simulink library "imu_block"  (R2025b)
settings: Solver=VariableStepAuto  StartTime=0.0  StopTime=10.0  RelTol=1e-3
values from neighbouring files (symbols this model uses):
  IMU_T03 = casper_imu_local_params()    [test_imu_model.m]
undefined symbols (not defined in the file or in its folder): ADXL, Attitude, Estimator, IMU, Sim
settings Model: Creator=Ashwin  LastModifiedBy=Ashwin

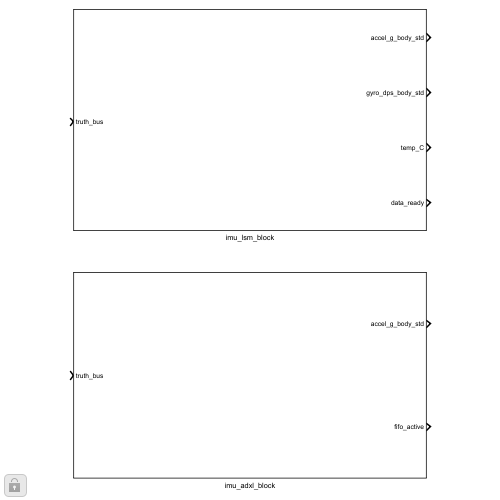
[thumbnail: Simulink's stored preview of the top-level diagram]
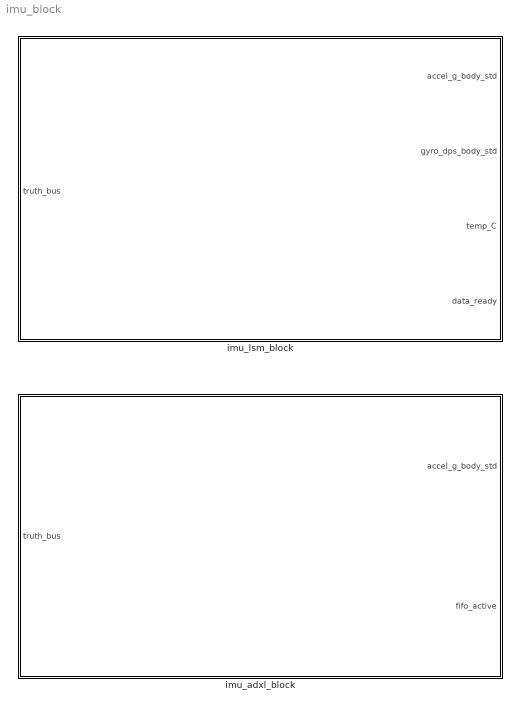
== system imu_block ==
  imu_adxl_block : Subsystem
  imu_lsm_block : Subsystem

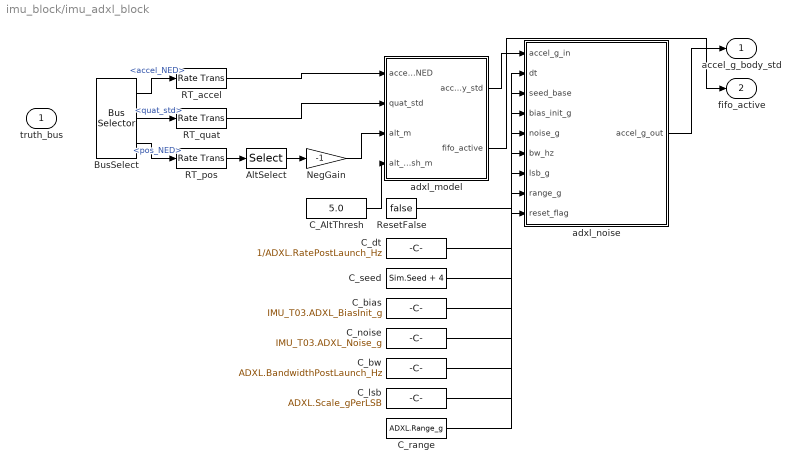
== system imu_block/imu_adxl_block ==
  truth_bus : Inport  OutDataTypeStr=Bus: TruthBus
  AltSelect : Selector  InputPortWidth=3  IndexOptions=Index vector (dialog)  Indices=3  OutputSizes=1
  BusSelect : BusSelector  OutputSignals=accel_NED,quat_std,pos_NED
  C_AltThresh : Constant  Value=5.0  SampleTime=1/ADXL.RatePostLaunch_Hz
  C_bias : Constant  Value=IMU_T03.ADXL_BiasInit_g  SampleTime=1/ADXL.RatePostLaunch_Hz
  C_bw : Constant  Value=ADXL.BandwidthPostLaunch_Hz  SampleTime=1/ADXL.RatePostLaunch_Hz
  C_dt : Constant  Value=1/ADXL.RatePostLaunch_Hz  SampleTime=1/ADXL.RatePostLaunch_Hz
  C_lsb : Constant  Value=ADXL.Scale_gPerLSB  SampleTime=1/ADXL.RatePostLaunch_Hz
  C_noise : Constant  Value=IMU_T03.ADXL_Noise_g  SampleTime=1/ADXL.RatePostLaunch_Hz
  C_range : Constant  Value=ADXL.Range_g  SampleTime=1/ADXL.RatePostLaunch_Hz
  C_seed : Constant  Value=Sim.Seed + 4  SampleTime=1/ADXL.RatePostLaunch_Hz
  NegGain : Gain  Gain=-1
  RT_accel : RateTransition  OutPortSampleTime=1/ADXL.RatePostLaunch_Hz
  RT_pos : RateTransition  OutPortSampleTime=1/ADXL.RatePostLaunch_Hz
  RT_quat : RateTransition  OutPortSampleTime=1/ADXL.RatePostLaunch_Hz
  ResetFalse : Constant  Value=false  OutDataTypeStr=boolean  SampleTime=1/ADXL.RatePostLaunch_Hz
  adxl_model : MATLAB Function  TreatAsAtomicUnit=on
  adxl_noise : MATLAB Function  TreatAsAtomicUnit=on
  accel_g_body_std : Outport
  fifo_active : Outport  Port=2
  wires:
  BusSelect/1 -> RT_accel/1  "<accel_NED>"
  BusSelect/2 -> RT_quat/1  "<quat_std>"
  BusSelect/3 -> RT_pos/1  "<pos_NED>"
  RT_pos/1 -> AltSelect/1
  AltSelect/1 -> NegGain/1
  RT_accel/1 -> adxl_model/1(accel_NED)
  RT_quat/1 -> adxl_model/2(quat_std)
  NegGain/1 -> adxl_model/3(alt_m)
  C_AltThresh/1 -> adxl_model/4(alt_launch_thresh_m)
  adxl_model/1(accel_g_body_std) -> adxl_noise/1(accel_g_in)
  C_dt/1 -> adxl_noise/2(dt)
  C_seed/1 -> adxl_noise/3(seed_base)
  C_bias/1 -> adxl_noise/4(bias_init_g)
  C_noise/1 -> adxl_noise/5(noise_g)
  C_bw/1 -> adxl_noise/6(bw_hz)
  C_lsb/1 -> adxl_noise/7(lsb_g)
  C_range/1 -> adxl_noise/8(range_g)
  ResetFalse/1 -> adxl_noise/9(reset_flag)
  adxl_noise/1(accel_g_out) -> accel_g_body_std/1
  adxl_model/2(fifo_active) -> fifo_active/1

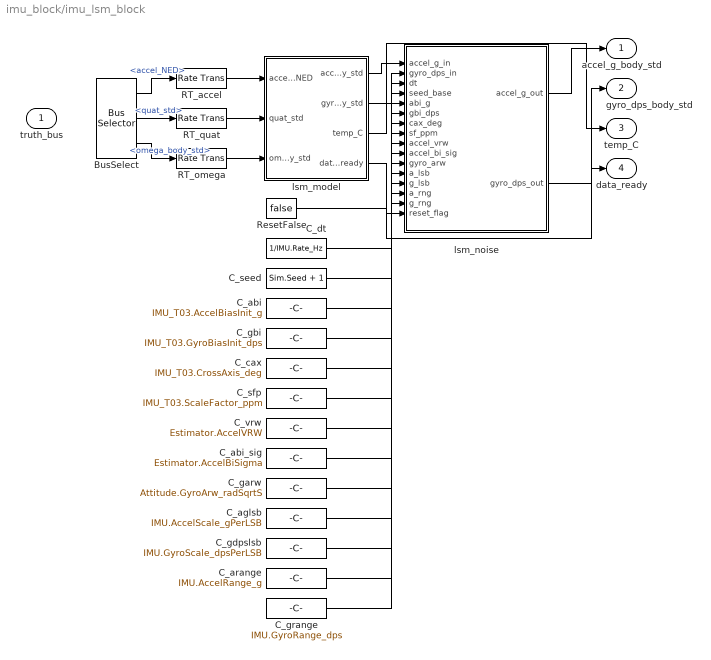
== system imu_block/imu_lsm_block ==
  truth_bus : Inport  OutDataTypeStr=Bus: TruthBus
  BusSelect : BusSelector  OutputSignals=accel_NED,quat_std,omega_body_std
  C_abi : Constant  Value=IMU_T03.AccelBiasInit_g  SampleTime=1/833
  C_abi_sig : Constant  Value=Estimator.AccelBiSigma  SampleTime=1/833
  C_aglsb : Constant  Value=IMU.AccelScale_gPerLSB  SampleTime=1/833
  C_arange : Constant  Value=IMU.AccelRange_g  SampleTime=1/833
  C_cax : Constant  Value=IMU_T03.CrossAxis_deg  SampleTime=1/833
  C_dt : Constant  Value=1/IMU.Rate_Hz  SampleTime=1/833
  C_garw : Constant  Value=Attitude.GyroArw_radSqrtS  SampleTime=1/833
  C_gbi : Constant  Value=IMU_T03.GyroBiasInit_dps  SampleTime=1/833
  C_gdpslsb : Constant  Value=IMU.GyroScale_dpsPerLSB  SampleTime=1/833
  C_grange : Constant  Value=IMU.GyroRange_dps  SampleTime=1/833
  C_seed : Constant  Value=Sim.Seed + 1  SampleTime=1/833
  C_sfp : Constant  Value=IMU_T03.ScaleFactor_ppm  SampleTime=1/833
  C_vrw : Constant  Value=Estimator.AccelVRW  SampleTime=1/833
  RT_accel : RateTransition  OutPortSampleTime=1/833
  RT_omega : RateTransition  OutPortSampleTime=1/833
  RT_quat : RateTransition  OutPortSampleTime=1/833
  ResetFalse : Constant  Value=false  OutDataTypeStr=boolean  SampleTime=1/833
  lsm_model : MATLAB Function  TreatAsAtomicUnit=on
  lsm_noise : MATLAB Function  TreatAsAtomicUnit=on
  accel_g_body_std : Outport
  gyro_dps_body_std : Outport  Port=2
  temp_C : Outport  Port=3
  data_ready : Outport  Port=4
  wires:
  BusSelect/1 -> RT_accel/1  "<accel_NED>"
  BusSelect/2 -> RT_quat/1  "<quat_std>"
  BusSelect/3 -> RT_omega/1  "<omega_body_std>"
  RT_accel/1 -> lsm_model/1(accel_NED)
  RT_quat/1 -> lsm_model/2(quat_std)
  RT_omega/1 -> lsm_model/3(omega_body_std)
  lsm_model/1(accel_g_body_std) -> lsm_noise/1(accel_g_in)
  lsm_model/2(gyro_dps_body_std) -> lsm_noise/2(gyro_dps_in)
  C_dt/1 -> lsm_noise/3(dt)
  C_seed/1 -> lsm_noise/4(seed_base)
  C_abi/1 -> lsm_noise/5(abi_g)
  C_gbi/1 -> lsm_noise/6(gbi_dps)
  C_cax/1 -> lsm_noise/7(cax_deg)
  C_sfp/1 -> lsm_noise/8(sf_ppm)
  C_vrw/1 -> lsm_noise/9(accel_vrw)
  C_abi_sig/1 -> lsm_noise/10(accel_bi_sig)
  C_garw/1 -> lsm_noise/11(gyro_arw)
  C_aglsb/1 -> lsm_noise/12(a_lsb)
  C_gdpslsb/1 -> lsm_noise/13(g_lsb)
  C_arange/1 -> lsm_noise/14(a_rng)
  C_grange/1 -> lsm_noise/15(g_rng)
  ResetFalse/1 -> lsm_noise/16(reset_flag)
  lsm_noise/1(accel_g_out) -> accel_g_body_std/1
  lsm_noise/2(gyro_dps_out) -> gyro_dps_body_std/1
  lsm_model/3(temp_C) -> temp_C/1
  lsm_model/4(data_ready) -> data_ready/1

== matlab function imu_block/imu_lsm_block/lsm_noise ==
  data: accel_g_in input; accel_g_out output; gyro_dps_in input; dt input; seed_base input; abi_g input; gbi_dps input; cax_deg input; sf_ppm input; accel_vrw input; accel_bi_sig input; gyro_arw input; a_lsb input; g_lsb input; a_rng input; g_rng input; reset_flag input; gyro_dps_out output
function [accel_g_out, gyro_dps_out] = fcn(accel_g_in, gyro_dps_in, dt, seed_base, abi_g, gbi_dps, cax_deg, sf_ppm, accel_vrw, accel_bi_sig, gyro_arw, a_lsb, g_lsb, a_rng, g_rng, reset_flag)
%#codegen
[accel_g_out, gyro_dps_out] = casper_imu_lsm_noise(accel_g_in, gyro_dps_in, dt, seed_base, abi_g, gbi_dps, cax_deg, sf_ppm, accel_vrw, accel_bi_sig, gyro_arw, a_lsb, g_lsb, a_rng, g_rng, reset_flag);
end

== matlab function imu_block/imu_lsm_block/lsm_model ==
  data: accel_NED input; accel_g_body_std output; quat_std input; omega_body_std input; gyro_dps_body_std output; temp_C output; data_ready output
function [accel_g_body_std, gyro_dps_body_std, temp_C, data_ready] = fcn(accel_NED, quat_std, omega_body_std)
%#codegen
[accel_g_body_std, gyro_dps_body_std, temp_C, data_ready] = casper_imu_lsm_model(accel_NED, quat_std, omega_body_std);
end

== matlab function imu_block/imu_adxl_block/adxl_model ==
  data: accel_NED input; accel_g_body_std output; quat_std input; alt_m input; alt_launch_thresh_m input; fifo_active output
function [accel_g_body_std, fifo_active] = fcn(accel_NED, quat_std, alt_m, alt_launch_thresh_m)
%#codegen
[accel_g_body_std, fifo_active] = casper_imu_adxl_model(accel_NED, quat_std, alt_m, alt_launch_thresh_m);
end

== matlab function imu_block/imu_adxl_block/adxl_noise ==
  data: accel_g_in input; accel_g_out output; dt input; seed_base input; bias_init_g input; noise_g input; bw_hz input; lsb_g input; range_g input; reset_flag input
function accel_g_out = fcn(accel_g_in, dt, seed_base, bias_init_g, noise_g, bw_hz, lsb_g, range_g, reset_flag)
%#codegen
accel_g_out = casper_imu_adxl_noise(accel_g_in, dt, seed_base, bias_init_g, noise_g, bw_hz, lsb_g, range_g, reset_flag);
end
